simulink model "MIP_Classicalcontroller"  (R2020b)
settings: Solver=VariableStepAuto  StartTime=0.0  StopTime=5  RelTol=1e-3
values from neighbouring files (symbols this model uses):
  A = [-(a+b)*j*XX (a+b)*j*XX a*d*XX;(b+c)*j*XX -(b+c)*j*XX -b*d*XX;1 0 0]    [Parameters.m]
  B = [-(a+b)*e*XX; (b+c)*e*XX; 0]    [Parameters.m]
  C = [1 0 0;0 1 0;0 0 1]    [Parameters.m]
  D = [0;0;0]    [Parameters.m]
settings Model: Creator=arthur  LastModifiedBy=arthur

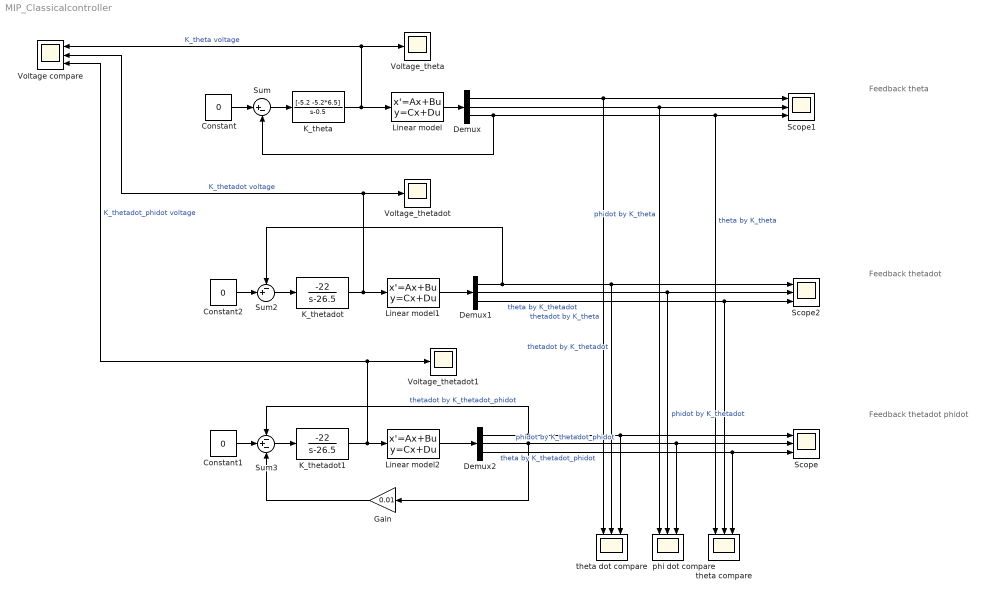
== system MIP_Classicalcontroller ==
  note: Feedback theta
  note: Feedback thetadot
  note: Feedback thetadot
      | phidot
  Constant : Constant  Value=0
  Constant1 : Constant  Value=0
  Constant2 : Constant  Value=0
  Demux : Demux  Outputs=3
  Demux1 : Demux  Outputs=3
  Demux2 : Demux  Outputs=3
  Gain : Gain  Gain=0.01
  K_theta : TransferFcn  Numerator=[-5.2 -5.2*6.5]  Denominator=[1 -0.5]
  K_thetadot : TransferFcn  Numerator=[-22]  Denominator=[1 -26.5]
  K_thetadot1 : TransferFcn  Numerator=[-22]  Denominator=[1 -26.5]
  Linear model : StateSpace  A=A  B=B  C=C  D=D  InitialCondition=[0 0 72*pi/180]
  Linear model1 : StateSpace  A=A  B=B  C=C  D=D  InitialCondition=[0 0 34*pi/180]
  Linear model2 : StateSpace  A=A  B=B  C=C  D=D  InitialCondition=[0 0 31*pi/180]
  Scope : Scope  NumInputPorts=3
  Scope1 : Scope  NumInputPorts=3
  Scope2 : Scope  NumInputPorts=3
  Sum : Sum  Inputs=|+-
  Sum2 : Sum  Inputs=-+|
  Sum3 : Sum  Inputs=-+-
  Voltage compare : Scope  NumInputPorts=3
  Voltage_theta : Scope
  Voltage_thetadot : Scope
  Voltage_thetadot1 : Scope
  phi dot compare : Scope  NumInputPorts=3
  theta compare : Scope  NumInputPorts=3
  theta dot compare : Scope  NumInputPorts=3
  wires:
  Demux/1 -> Scope1/1, theta dot compare/1  "thetadot by K_theta"
  Demux/3 -> Sum/2, theta compare/1, Scope1/3  "theta by K_theta"
  Demux/2 -> phi dot compare/1, Scope1/2  "phidot by K_theta"
  Constant/1 -> Sum/1
  Sum/1 -> K_theta/1
  Linear model/1 -> Demux/1
  K_theta/1 -> Voltage compare/1, Voltage_theta/1, Linear model/1  "K_theta voltage"
  K_thetadot/1 -> Linear model1/1, Voltage compare/2, Voltage_thetadot/1  "K_thetadot voltage"
  Sum2/1 -> K_thetadot/1
  Demux1/1 -> Sum2/1, Scope2/1, theta dot compare/2  "thetadot by K_thetadot"
  Demux1/2 -> Scope2/2, phi dot compare/2  "phidot by K_thetadot"
  Demux1/3 -> Scope2/3, theta compare/2  "theta by K_thetadot"
  Linear model1/1 -> Demux1/1
  Constant2/1 -> Sum2/2
  K_thetadot1/1 -> Linear model2/1, Voltage compare/3, Voltage_thetadot1/1  "K_thetadot_phidot voltage"
  Linear model2/1 -> Demux2/1
  Demux2/2 -> phi dot compare/3, Scope/2, Gain/1  "phidot by K_thetadot_phidot"
  Demux2/1 -> Scope/1, theta dot compare/3, Sum3/1  "thetadot by K_thetadot_phidot"
  Demux2/3 -> theta compare/3, Scope/3  "theta by K_thetadot_phidot"
  Sum3/1 -> K_thetadot1/1
  Constant1/1 -> Sum3/2
  Gain/1 -> Sum3/3
